simulink model "robotmove1meter"  (R2023a)
settings: Solver=FixedStepDiscrete  StartTime=0.0  StopTime=30  FixedStep=0.01  RelTol=1e-3
undefined symbols (not defined in the file or in its folder): ticksPerRot, wheelR
libraries: mobileRoboticsTrainingLib x3
settings Model: Creator=Boitumelo  LastModifiedBy=thuto
settings DebuggingCC: UnconnectedInputMsg=warning  UnconnectedOutputMsg=warning  UnconnectedLineMsg=warning
settings ModelReferenceCC: EnableRefExpFcnMdlSchedulingChecks=on
settings RTWCC: DLArmComputeVersion=19.05

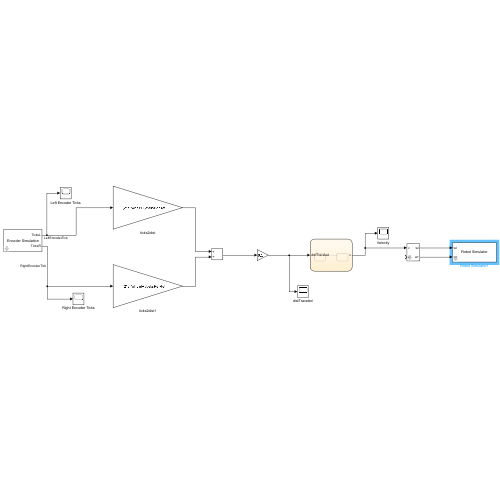
[thumbnail: Simulink's stored preview of the top-level diagram]
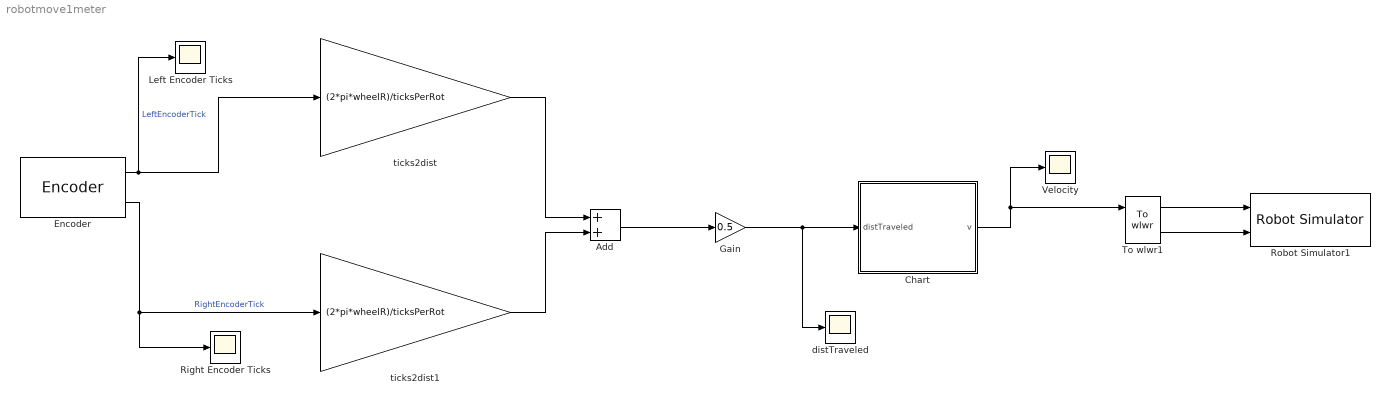
== system robotmove1meter ==
  Add : Sum
  Chart : Stateflow chart  TreatAsAtomicUnit=on
  Encoder : mobileRoboticsTrainingLib/Encoder  axleLength=axleLength  wheelR=wheelR  ticksPerRot=ticksPerRot
      settings: SourceProductName=Mobile Robotics Training Library
  Gain : Gain  Gain=0.5
  Left Encoder Ticks : Scope
  Right Encoder Ticks : Scope
  Robot Simulator1 : mobileRoboticsTrainingLib/Robot Simulator  Priority=99  mapVar=mapForSim  startX=0.5  startY=0.1  startTheta=90  axleLength=axleLength  wheelR=wheelR
  To wlwr1 : mobileRoboticsTrainingLib/To wlwr  axleLength=0.1  wheelR=0.05
  Velocity : Scope
  distTraveled : Scope
  ticks2dist : Gain  Gain=(2*pi*wheelR)/ticksPerRot
  ticks2dist1 : Gain  Gain=(2*pi*wheelR)/ticksPerRot
  wires:
  Encoder/1 -> ticks2dist/1, Left Encoder Ticks/1  "LeftEncoderTick"
  Encoder/2 -> Right Encoder Ticks/1, ticks2dist1/1  "RightEncoderTick"
  ticks2dist/1 -> Add/1
  ticks2dist1/1 -> Add/2
  Add/1 -> Gain/1
  Gain/1 -> distTraveled/1, Chart/1(distTraveled)
  Chart/1(v) -> To wlwr1/1, Velocity/1
  To wlwr1/1 -> Robot Simulator1/1
  To wlwr1/2 -> Robot Simulator1/2

== stateflow chart robotmove1meter/Chart ==
  state MoveForward
    entry: v=0.1
  state Stop
    entry: v=0
  (default) -> MoveForward
  MoveForward -> Stop : [distTraveled >= 1]
  data: distTraveled input; v output
